simulink model "W01_P1"  (R2024b)
settings: Solver=ode4  StartTime=0  StopTime=T_final  FixedStep=h  RelTol=1e-3
undefined symbols (not defined in the file or in its folder): beta_c, mp, rp, V_c, x0
settings Model: Creator=admin  LastModifiedBy=admin
settings DataIOCC: ReturnWorkspaceOutputs=off

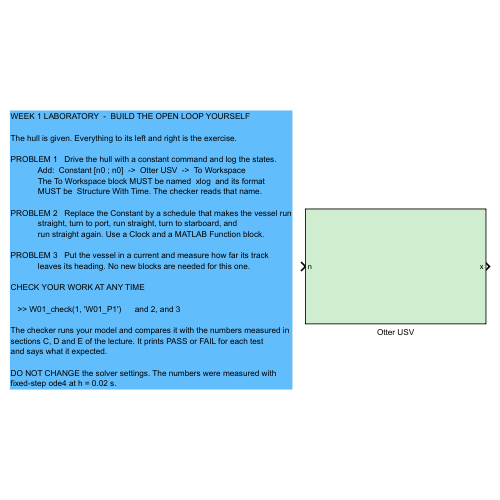
[thumbnail: Simulink's stored preview of the top-level diagram]
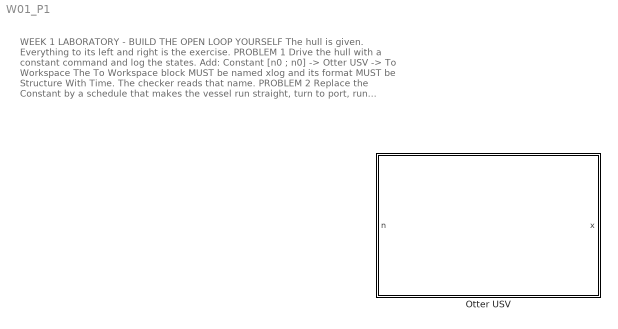
== system W01_P1 ==
  note: WEEK 1 LABORATORY  -  BUILD THE OPEN LOOP YOURSELF
      |
      | The hull is given. Everything to its left and right is the exercise.
      |
      | PROBLEM 1   Drive the hull with a constant command and log the states.
      |             Add:  Constant [n0 ; n0]  ->  Otter USV  ->  To Workspace
      |             The To Workspace block MUST be named  xlog  and its format
      |             MUST be  Structure With Time. The checker reads that name.
      |
      | PROBLEM 2   Replace the Constant by a schedule that makes the vessel run
      |             straight, turn to port, run straight, turn to starboard, and
      |             run straight again. Use a Clock and a MATLAB Function block.
      |
      | PROBLEM 3   Put the vessel in a current and measure how far its track
      |             leaves its heading. No new blocks are needed for this one.
      |
      | CHECK YOUR WORK AT ANY TIME
      |
      |    >> W01_check(1, 'W01_P1')      and 2, and 3
      |
      | The checker runs your model and compares it with the numbers measured in
      | sections C, D and E of the lecture. It prints PASS or FAIL for each test
      | and says what it expected.
      |
      | DO NOT CHANGE the solver settings. The numbers were measured with
      | fixed-step ode4 at h = 0.02 s.
  Otter USV : Subsystem

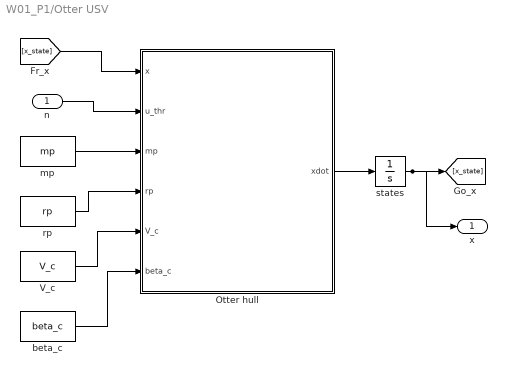
== system W01_P1/Otter USV ==
  n : Inport
  Otter hull : MATLAB Function  TreatAsAtomicUnit=on
  V_c : Constant  Value=V_c
  beta_c : Constant  Value=beta_c
  mp : Constant  Value=mp
  rp : Constant  Value=rp
  states : Integrator  InitialCondition=x0
  x : Outport
  wires:
  beta_c/1 -> Otter hull/6(beta_c)
  [x_state] -> Otter hull/1(x)
  rp/1 -> Otter hull/4(rp)
  n/1 -> Otter hull/2(u_thr)
  mp/1 -> Otter hull/3(mp)
  V_c/1 -> Otter hull/5(V_c)
  states/1 -> [x_state], x/1
  Otter hull/1(xdot) -> states/1

== matlab function W01_P1/Otter USV/Otter hull ==
  data: x input; xdot output double size=[12 1]; u_thr input; mp input; rp input; V_c input; beta_c input
function xdot = otter_hull(x, u_thr, mp, rp, V_c, beta_c)
% Fossen's otter.m, called unchanged from Tools/MSS/VESSELS.
%
%   x       12 states, fed back from the integrator
%   u_thr   propeller shaft speeds [rad/s]
%
% otter.m is not written for code generation, so the call is extrinsic and
% xdot has to be pre-sized for Simulink to know the output width.
coder.extrinsic('otter');

xdot = zeros(12,1);
xdot = otter(x, u_thr, mp, rp, V_c, beta_c);
end
